simulink model "block"  (R2013b)
settings: Solver=ode45  StartTime=0.0  StopTime=Inf  RelTol=1e-3
settings Model: Creator=Bing  LastModifiedBy=geyer_adm
settings DataIOCC: SignalLoggingSaveFormat=ModelDataLogs
settings DebuggingCC: UnderspecifiedInitializationDetection=Simplified  MultiTaskDSMMsg=warning  MultiTaskCondExecSysMsg=none
settings RTWCC: IncludeERTFirstTime=on
settings GRTTargetCC: CodeReplacementLibrary=None  CPPClassGenCompliant=on

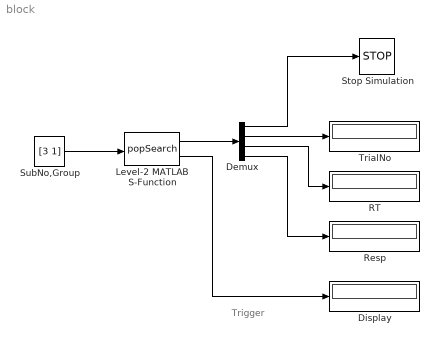
== system block ==
  note: Trigger
  Demux : Demux
  Display : Display
  Level-2 MATLAB S-Function : M-S-Function  FunctionName=popSearch
  RT : Display
  Resp : Display
  Stop Simulation : Stop
  SubNo,Group : Constant  Value=[3 1]
  TrialNo : Display
  wires:
  SubNo,Group/1 -> Level-2 MATLAB S-Function/1
  Level-2 MATLAB S-Function/1 -> Demux/1
  Demux/4 -> Resp/1
  Demux/3 -> RT/1
  Demux/2 -> TrialNo/1
  Demux/1 -> Stop Simulation/1
  Level-2 MATLAB S-Function/2 -> Display/1
